simulink model "model_bf"  (Simulink 6.3)
settings: Solver=ode45  StartTime=0.0  StopTime=10.0  RelTol=1e-3
libraries: cstblocks x2
settings Model: Creator=fromion  LastModifiedBy=anne  ExtModeTrigMode=oneshot  ExtModeArmWhenConnect=off  ExtModeAutoUpdateStatusClock=off
settings DataIOCC: LimitDataPoints=off
settings OptimizationCC: BlockReduction=off  BooleanDataType=off
settings DebuggingCC: SolverPrmCheckMsg=none
settings HardwareCC: TargetUnknown=on
settings GRTTargetCC: TargetFcnLib=ansi_tfl_table_tmw.mat  ModelReferenceCompliant=off  MatFileLogging=off

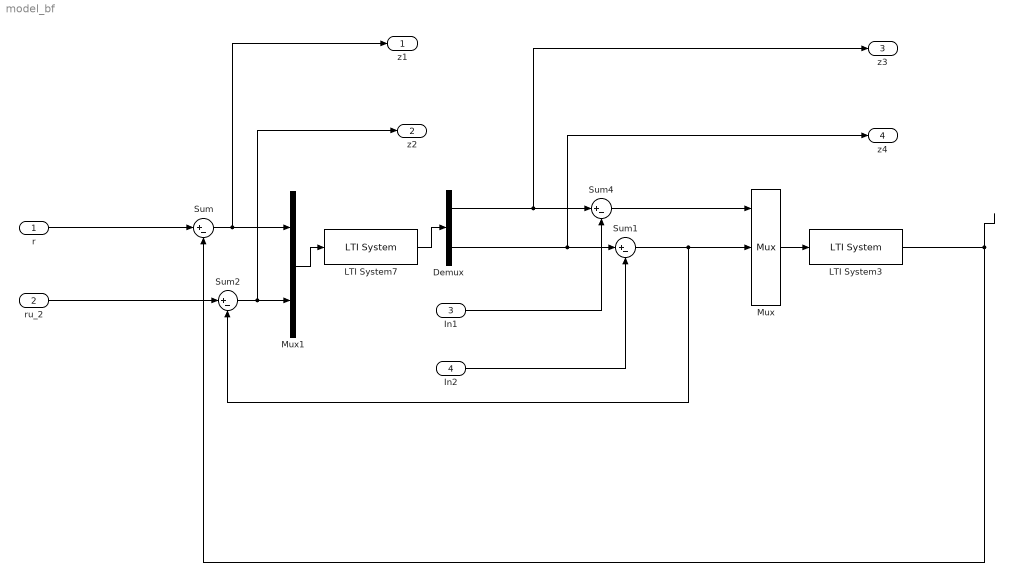
== system model_bf ==
  r : Inport  OutDataType=fixdt(1,16,0)  OutScaling=[]
  ru_2 : Inport  Port=2  OutDataType=fixdt(1,16,0)  OutScaling=[]
  In1 : Inport  Port=3  OutDataType=fixdt(1,16,0)  OutScaling=[]
  In2 : Inport  Port=4  OutDataType=fixdt(1,16,0)  OutScaling=[]
  Demux : Demux  Outputs=2
  LTI System3 : cstblocks/LTI System  sys=sys_synt_ss  IC=0
  LTI System7 : cstblocks/LTI System  sys=K_hinf_ss  IC=0
  Mux : Mux  Inputs=3
  Mux1 : Mux  Inputs=2
  Sum{,1..2,4} (4 alike) : Sum  Inputs=|+-  OutDataType=fixdt(1,16,0)  OutScaling=[]  SaturateOnIntegerOverflow=on  InputSameDT=on
  z1 : Outport  OutDataType=fixdt(1,16,0)  OutScaling=[]
  z2 : Outport  Port=2  OutDataType=fixdt(1,16,0)  OutScaling=[]
  z3 : Outport  Port=3  OutDataType=fixdt(1,16,0)  OutScaling=[]
  z4 : Outport  Port=4  OutDataType=fixdt(1,16,0)  OutScaling=[]
  wires:
  Sum/1 -> Mux1/1, z1/1
  In1/1 -> Sum4/2
  r/1 -> Sum/1
  LTI System3/1 -> Sum/2
  Sum4/1 -> Mux/1
  Demux/2 -> Sum1/1, z4/1
  Sum1/1 -> Sum2/2, Mux/2
  In2/1 -> Sum1/2
  ru_2/1 -> Sum2/1
  Sum2/1 -> Mux1/2, z2/1
  Mux/1 -> LTI System3/1
  Demux/1 -> Sum4/1, z3/1
  Mux1/1 -> LTI System7/1
  LTI System7/1 -> Demux/1
